simulink model "nonlinear_ss_control_reg_obs"  (R2019b)
settings: Solver=ode45  StartTime=0.0  StopTime=16600  MaxStep=0.001  RelTol=1e-8
settings Model: Creator=Hector  LastModifiedBy=Hector

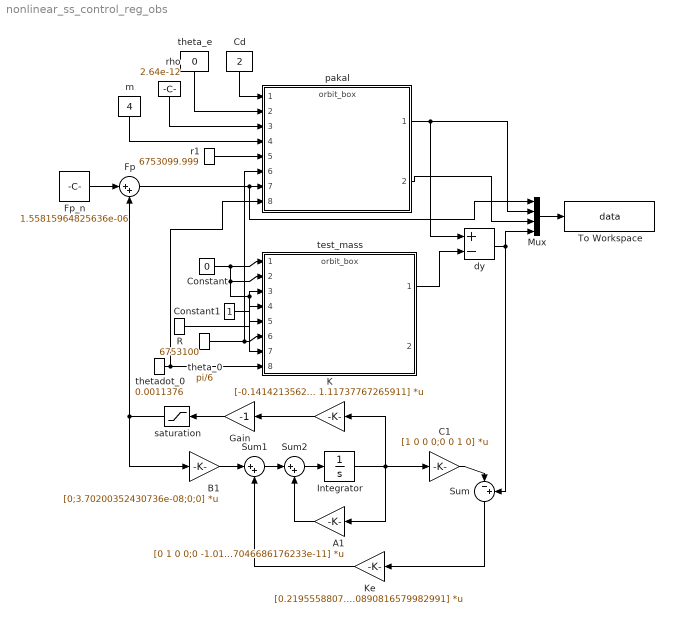
== system nonlinear_ss_control_reg_obs ==
  A1 : Gain  Gain=[0 1 0 0;0 -1.01409337235247e-10 -1.70834505909243e-20 -3.36920663455173e-10;0 0 0 1;0 15365.0510962495 3.88260240702825e-06 -5.07046686176233e-11]  Multiplication=Matrix(K*u)
  B1 : Gain  Gain=[0;3.70200352430736e-08;0;0]  Multiplication=Matrix(K*u)
  C1 : Gain  Gain=[1 0 0 0;0 0 1 0]  Multiplication=Matrix(K*u)
  Cd : Constant  Value=2
  Constant : Constant  Value=0
  Constant1 : Constant
  Fp : Sum  Inputs=|++
  Fp_n : Constant  Value=1.55815964825636e-06
  Gain : Gain  Gain=-1
  Integrator : Integrator  InitialCondition=[0, 0, -1*10^-3, 0].'
  K : Gain  Gain=[-0.141421356249834 963078.733398081 0.010243364845765 1.11737767265911]  Multiplication=Matrix(K*u)
  Ke : Gain  Gain=[0.219555880769803 -6.20274847519216e-06;0.0115827344660038 -5.53693888523524e-07;13913.3056289779 0.159444119063664;3243.30558114425 -0.0890816579982991]  Multiplication=Matrix(K*u)
  Mux : Mux
  R : Constant  Value=6753100
  Sum : Sum  Inputs=|-+
  Sum1 : Sum  Inputs=|++
  Sum2 : Sum  Inputs=|++
  To Workspace : ToWorkspace  VariableName=data  SaveFormat=Timeseries  SampleTime=-1
  dy : Sum  Inputs=+-
  m : Constant  Value=4
  pakal : ModelReference  ModelNameDialog=orbit_box.slx  SimulationMode=Normal  ModelReferenceVersion=1.40
  r1 : Constant  Value=6753099.999
  rho : Constant  Value=2.64e-12
  saturation : Saturate  UpperLimit=1.8442e-05  LowerLimit=-1.5582e-06
  test_mass : ModelReference  ModelNameDialog=orbit_box.slx  SimulationMode=Normal  ModelReferenceVersion=1.40
  theta_0 : Constant  Value=pi/6
  theta_e : Constant  Value=0
  thetadot_0 : Constant  Value=0.0011376
  wires:
  Fp_n/1 -> Fp/1
  R/1 -> test_mass/5
  Constant1/1 -> test_mass/4
  r1/1 -> pakal/5
  m/1 -> pakal/4
  rho/1 -> pakal/3
  theta_e/1 -> pakal/2
  Cd/1 -> pakal/1
  Mux/1 -> To Workspace/1
  K/1 -> Gain/1
  theta_0/1 -> pakal/6, test_mass/6
  Constant/1 -> test_mass/7, test_mass/3, test_mass/2, test_mass/1
  pakal/1 -> dy/1, Mux/2
  pakal/2 -> Mux/3
  thetadot_0/1 -> pakal/8, test_mass/8
  Sum2/1 -> Integrator/1
  Integrator/1 -> K/1, C1/1, A1/1
  Ke/1 -> Sum1/2
  B1/1 -> Sum1/1
  A1/1 -> Sum2/2
  saturation/1 -> Fp/2, B1/1
  C1/1 -> Sum/1
  Sum/1 -> Ke/1
  Sum1/1 -> Sum2/1
  dy/1 -> Sum/2, Mux/4
  test_mass/1 -> dy/2
  Fp/1 -> Mux/1, pakal/7
  Gain/1 -> saturation/1
